simulink model "MotorModelFullCopy"  (R2020b)
settings: Solver=ode45  StartTime=0.0  StopTime=13  RelTol=1e-3  EnableMultiTasking=on
PreLoadFcn:
  | MotorParam
InitFcn:
  | MotorParam
values from neighbouring files (symbols this model uses):
  Ampden1 = [1 7179 3.552e07]    [FullProjectMatlabCode.m]
  Ampden2 = [1 7243 3.59e07]    [FullProjectMatlabCode.m]
  Ampden3 = [1 1.475e04 1.91e08]    [FullProjectMatlabCode.m]
  Ampnum1 = [8.029e07]    [FullProjectMatlabCode.m]
  Ampnum2 = [8.126e07]    [FullProjectMatlabCode.m]
  Ampnum3 = [1.412e08]    [FullProjectMatlabCode.m]
  Kb1 = 1/((494*pi)/30)    (= 0.0193305598897)    [FullProjectMatlabCode.m]
  Kb2 = 1/((637*pi)/30)    (= 0.0149910464451)    [FullProjectMatlabCode.m]
  Kb3 = 1/((3310*pi)/30)    (= 0.00288498386269)    [FullProjectMatlabCode.m]
  Km1 = 19.3e-3    (= 0.0193)    [FullProjectMatlabCode.m]
  Km2 = 15.0e-3    (= 0.015)    [FullProjectMatlabCode.m]
  Km3 = 2.16e-3    (= 0.00216)    [FullProjectMatlabCode.m]
  L1 = 0.413e-3    (= 0.000413)    [FullProjectMatlabCode.m]
  L2 = 0.610e-03    (= 0.00061)    [FullProjectMatlabCode.m]
  L3 = 0.363e-3    (= 0.000363)    [FullProjectMatlabCode.m]
  R1 = 6.28    [FullProjectMatlabCode.m]
  R2 = 19.1    [FullProjectMatlabCode.m]
  R3 = 37.2    [FullProjectMatlabCode.m]
libraries: simulink x4
settings Model: Creator=Leo  LastModifiedBy=Mibo
settings DataIOCC: LimitDataPoints=on  SaveFormat=Array  SignalLoggingSaveFormat=ModelDataLogs  ReturnWorkspaceOutputs=off
settings OptimizationCC: ExpressionDepthLimit=2147483647  InitFltsAndDblsToZero=on  LifeSpan=inf
settings DebuggingCC: UnderspecifiedInitializationDetection=Classic  MergeDetectMultiDrivingBlocksExec=none  SolverPrmCheckMsg=warning  FcnCallInpInsideContextMsg=warning  StateNameClashWarn=warning  SFUnexpectedBacktrackingDiag=warning  SFNoUnconditionalDefaultTransitionDiag=warning  SFExecutionAtInitializationDiag=none  ArithmeticOperatorsInVariantConditions=warning
settings HardwareCC: ProdBitPerPointer=32  ProdBitPerSizeT=32  ProdBitPerPtrDiffT=32  ProdLargestAtomicFloat=None  ProdIntDivRoundTo=Undefined  ProdEndianess=Unspecified  ProdWordSize=32  ProdHWDeviceType=32-bit Generic
settings ModelReferenceCC: PropagateSignalLabelsOutOfModel=off
settings SFSimCC: SimUseLocalCustomCode=off  CustomCodeUndefinedFunction=UseInterfaceOnly
settings RTWCC: RTWUseLocalCustomCode=off
settings CodeAppCC: StateflowObjectComments=on
settings GRTTargetCC: TargetLangStandard=C89/C90 (ANSI)  CombineOutputUpdateFcns=off  GRTInterface=on
settings ConfigComp: CovMetricSettings=dw  CovSaveCumulativeToWorkspaceVar=on  CovSaveSingleToWorkspaceVar=on  CovExternalEMLEnable=off  CovSFcnEnable=off

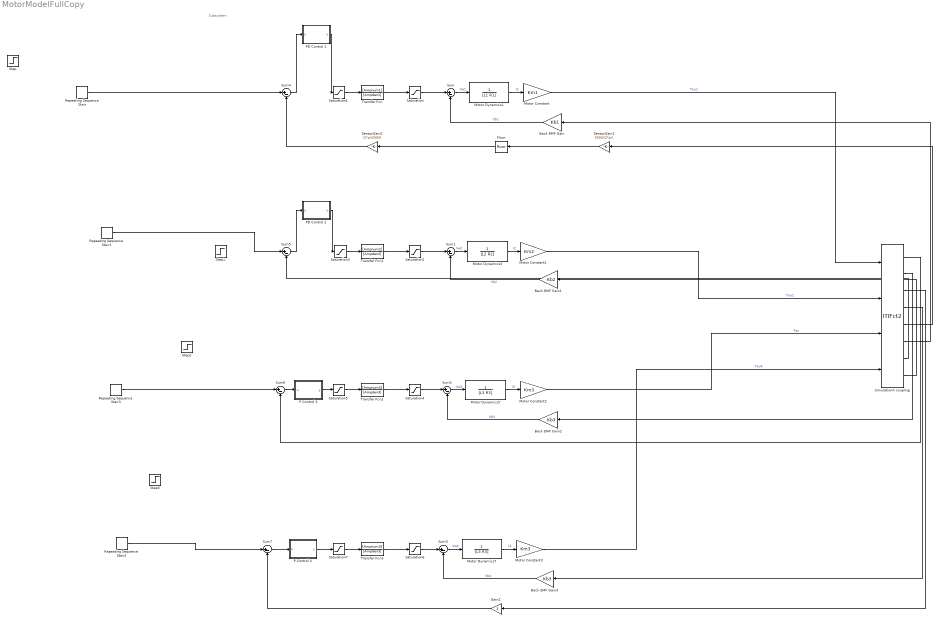
== system MotorModelFullCopy ==
  note: Subsystem
  Back EMF Gain : Gain  Gain=Kb1
  Back EMF Gain1 : Gain  Gain=Kb2
  Back EMF Gain2 : Gain  Gain=Kb3
  Back EMF Gain3 : Gain  Gain=Kb3
  Floor : Rounding
  Gain2 : Gain
  Motor Constant : Gain  Gain=Km1
  Motor Constant1 : Gain  Gain=Km2
  Motor Constant2 : Gain  Gain=Km3
  Motor Constant3 : Gain  Gain=Km3
  Motor Dynamics1 : TransferFcn  Denominator=[L1 R1]
  Motor Dynamics3 : TransferFcn  Denominator=[L2 R2]
  Motor Dynamics5 : TransferFcn  Denominator=[L3 R3]
  Motor Dynamics7 : TransferFcn  Denominator=[L3 R3]
  P Control 3 : MATLAB Function  TreatAsAtomicUnit=on
  P Control 4 : MATLAB Function  TreatAsAtomicUnit=on
  PD Control 1 : MATLAB Function  TreatAsAtomicUnit=on
  PD Control 2 : MATLAB Function  TreatAsAtomicUnit=on
  Repeating Sequence Stair : simulink/Sources/Repeating Sequence Stair  OutValues=A3  tsamp=1  OutMin=[]  OutMax=[]  OutDataTypeStr=double  OutputDataTypeScalingMode=double  OutDataType=fixdt(0,8)  ConRadixGroup=Best Precision: Vector-wise  OutScaling=2^-12
  Repeating Sequence Stair1 : simulink/Sources/Repeating Sequence Stair  OutValues=E3  tsamp=1  OutMin=[]  OutMax=[]  OutDataTypeStr=double  OutputDataTypeScalingMode=double  OutDataType=fixdt(0,8)  ConRadixGroup=Best Precision: Vector-wise  OutScaling=2^-12
  Repeating Sequence Stair2 : simulink/Sources/Repeating Sequence Stair  OutValues=G3  tsamp=1  OutMin=[]  OutMax=[]  OutDataTypeStr=double  OutputDataTypeScalingMode=double  OutDataType=fixdt(0,8)  ConRadixGroup=Best Precision: Vector-wise  OutScaling=2^-12
  Repeating Sequence Stair3 : simulink/Sources/Repeating Sequence Stair  OutValues=W3  tsamp=1  OutMin=[]  OutMax=[]  OutDataTypeStr=double  OutputDataTypeScalingMode=double  OutDataType=fixdt(0,8)  ConRadixGroup=Best Precision: Vector-wise  OutScaling=2^-12
  Saturation : Saturate  UpperLimit=12  LowerLimit=-12
  Saturation{1,3,5,7} (4 alike) : Saturate  UpperLimit=5  LowerLimit=-5
  Saturation2 : Saturate  UpperLimit=12  LowerLimit=-12
  Saturation4 : Saturate  UpperLimit=6  LowerLimit=-6
  Saturation6 : Saturate  UpperLimit=6  LowerLimit=-6
  SensorGain1 : Gain  Gain=5000/(2*pi)
  SensorGain2 : Gain  Gain=(2*pi)/5000
  SimulationX coupling : S-Function  FunctionName=ITIFct2  Parameters=ip, port, ts, nIn, nOut  SFunctionDeploymentMode=off  EnableBusSupport=off  mask{ip='localhost', port=4096, ts=0.001, nIn=4, nOut=8}
      mask prompts: ip "Address: ip"; port "Port Number: port [-]"; ts "Communication Step Size: ts [s]"; nIn "Input Vector Dimension (to SimulationX): nIn [-]"; nOut "Output Vector Dimension (from SimulationX): nOut [-]"
      mask help: Coupling Element
  Step : Step  Time=0.5  After=0.34907  SampleTime=1e-3
  Step1 : Step  Time=0.5  After=1.53589  SampleTime=1e-3
  Step2 : Step  Time=0.5  After=0  SampleTime=1e-3
  Step3 : Step  Time=0.5  After=0  SampleTime=1e-3
  Sum{,1..7} (8 alike) : Sum  Inputs=|+-
  Transfer Fcn : TransferFcn  Numerator=[Ampnum1]  Denominator=[Ampden1]
  Transfer Fcn1 : TransferFcn  Numerator=[Ampnum2]  Denominator=[Ampden2]
  Transfer Fcn2 : TransferFcn  Numerator=[Ampnum3]  Denominator=[Ampden3]
  Transfer Fcn3 : TransferFcn  Numerator=[Ampnum3]  Denominator=[Ampden3]
  wires:
  P Control 3/1(y) -> Saturation5/1
  Sum6/1 -> P Control 3/1(u)
  P Control 4/1(y) -> Saturation7/1
  Sum7/1 -> P Control 4/1(u)
  PD Control 2/1(y) -> Saturation3/1
  Sum5/1 -> PD Control 2/1(u)
  PD Control 1/1(y) -> Saturation1/1
  Sum4/1 -> PD Control 1/1(u)
  SimulationX coupling/4 -> Back EMF Gain3/1
  SimulationX coupling/3 -> Gain2/1
  SimulationX coupling/8 -> Back EMF Gain1/1
  SimulationX coupling/7 -> Sum5/2
  SimulationX coupling/1 -> Sum6/2
  SimulationX coupling/2 -> Back EMF Gain2/1
  SimulationX coupling/6 -> Back EMF Gain/1
  SimulationX coupling/5 -> SensorGain1/1
  Gain2/1 -> Sum7/2
  Motor Constant3/1 -> SimulationX coupling/4  "Tau4"
  Motor Constant2/1 -> SimulationX coupling/3  "Tau"
  Motor Constant1/1 -> SimulationX coupling/2  "Tau2"
  Motor Constant/1 -> SimulationX coupling/1  "Tau1"
  Floor/1 -> SensorGain2/1
  SensorGain2/1 -> Sum4/2
  SensorGain1/1 -> Floor/1
  Sum2/1 -> Motor Dynamics5/1  "Vw3"
  Transfer Fcn1/1 -> Saturation2/1
  Saturation7/1 -> Transfer Fcn3/1
  Motor Dynamics7/1 -> Motor Constant3/1  "I4"
  Saturation1/1 -> Transfer Fcn/1
  Saturation2/1 -> Sum1/1
  Saturation/1 -> Sum/1
  Saturation3/1 -> Transfer Fcn1/1
  Transfer Fcn/1 -> Saturation/1
  Transfer Fcn3/1 -> Saturation6/1
  Motor Dynamics5/1 -> Motor Constant2/1  "I3"
  Saturation4/1 -> Sum2/1
  Back EMF Gain/1 -> Sum/2  "Vb1"
  Sum1/1 -> Motor Dynamics3/1  "Vw2"
  Transfer Fcn2/1 -> Saturation4/1
  Sum/1 -> Motor Dynamics1/1  "Vw1"
  Sum3/1 -> Motor Dynamics7/1  "Vw4"
  Saturation5/1 -> Transfer Fcn2/1
  Back EMF Gain3/1 -> Sum3/2  "Vb4"
  Back EMF Gain1/1 -> Sum1/2  "Vb2"
  Back EMF Gain2/1 -> Sum2/2  "Vb3"
  Motor Dynamics3/1 -> Motor Constant1/1  "I2"
  Saturation6/1 -> Sum3/1
  Motor Dynamics1/1 -> Motor Constant/1  "I1"
  Repeating Sequence Stair/1 -> Sum4/1
  Repeating Sequence Stair1/1 -> Sum5/1
  Repeating Sequence Stair3/1 -> Sum6/1
  Repeating Sequence Stair2/1 -> Sum7/1

== matlab function MotorModelFullCopy/P Control 3 ==
  settings: updateMethod=DISCRETE  sampleTime=1e-3
  data: u input; y output
function y = fcn(u)
persistent previous
persistent weight
persistent temp
T = 1e-3;
Kp = 20;
Kd = 0.008;

if (isempty(previous))
    previous = zeros(1,10);
end

if (isempty(temp))
    temp = 0;
end

if (isempty(weight))
    weight = zeros(1,10);
    for n = 1:10
        weight(n) = 400*Kd*exp(-400*n*T)
    end
end

previous(1) = (u-temp)/T;
deriv = dot(weight,previous);

for n = 1:9
    previous(11-n) = previous(11-n-1);
end

temp = u;

output = Kp*u+deriv
    
y = output  ;

== matlab function MotorModelFullCopy/PD Control 2 ==
  settings: updateMethod=DISCRETE  sampleTime=1e-3
  data: u input; y output
function y = PDControl2(u)
persistent previous
persistent weight
persistent temp
T = 1e-3;
Kp = 25;
Kd = 0.0123;

if (isempty(previous))
    previous = zeros(1,10);
end

if (isempty(temp))
    temp = 0;
end

if (isempty(weight))
    weight = zeros(1,10);
    for n = 1:10
        weight(n) = 400*Kd*exp(-400*n*T)
    end
end

previous(1) = (u-temp)/T;
deriv = dot(weight,previous);

for n = 1:9
    previous(11-n) = previous(11-n-1);
end

temp = u;

output = Kp*u+deriv
    
y = output  ;

== matlab function MotorModelFullCopy/P Control 4 ==
  settings: updateMethod=DISCRETE  sampleTime=1e-3
  data: u input; y output
function y = PControl4(u)
persistent previous
persistent weight
persistent temp
T = 1e-3;
Kp = 20;
Kd = 0.008;

if (isempty(previous))
    previous = zeros(1,10);
end

if (isempty(temp))
    temp = 0;
end

if (isempty(weight))
    weight = zeros(1,10);
    for n = 1:10
        weight(n) = 400*Kd*exp(-400*n*T)
    end
end

previous(1) = (u-temp)/T;
deriv = dot(weight,previous);

for n = 1:9
    previous(11-n) = previous(11-n-1);
end

temp = u;

output = Kp*u+deriv
    
y = output  ;

== matlab function MotorModelFullCopy/PD Control 1 ==
  settings: updateMethod=DISCRETE  sampleTime=1e-3
  data: u input; y output
function y = PDControl1(u)
persistent previous
persistent weight
persistent temp
T = 1e-3;
Kp = 45;
Kd = 0.03;

if (isempty(previous))
    previous = zeros(1,10);
end

if (isempty(temp))
    temp = 0;
end

if (isempty(weight))
    weight = zeros(1,10);
    for n = 1:10
        weight(n) = 400*Kd*exp(-400*n*T)
    end
end

previous(1) = (u-temp)/T;
deriv = dot(weight,previous);

for n = 1:9
    previous(11-n) = previous(11-n-1);
end

temp = u;

output = Kp*u+deriv
    
y = output  ;
